simulink model "slexCreditRatingClassificationEnsemblePredictExample"  (R2021a)
settings: Solver=FixedStepDiscrete  StartTime=0.0  StopTime=creditRatingInput.time(end)  RelTol=1e-3
PreLoadFcn:
  | tbl = readtable('CreditRating_Historical.dat');
  | 
  | d = dummyvar(tbl.Industry);
  | X = [table2array(tbl(:,2:6)) d];
  | Y = tbl.Rating;
  | 
  | prsntX = X(1:3000,:);
  | prsntY = Y(1:3000);
  | ftrX = X(3001:end,:);
  | ftrY = Y(3001:end);
  | 
  | rng('default')
  | t = templateTree('Reproducible',true,'MinLeafSize',5);
  | ensMdl = fitcensemble(prsntX,prsntY, ...
  |     'Learners',t, ...
  |     'ClassNames',{'AAA' 'AA' 'A' 'BBB' 'BB' 'B' 'CCC'}, ...
  |     'Method','Bag', ...
  |     'NumLearningCycles',499');
  | 
  | creditRatingInput.time = (0:931)';
  | creditRatingInput.signals(1).values = ftrX;
  | creditRatingInput.signals(1).dimensions = size(ftrX,2);
libraries: statsLibrary x1
settings Model: Creator=The MathWorks, Inc.  LastModifiedBy=The MathWorks, Inc.
settings SolverCC: AlgebraicLoopSolver=TrustRegion
settings DataIOCC: ExternalInput=creditRatingInput  LoadExternalInput=on
settings DebuggingCC: SFMachineParentedDataDiag=warning

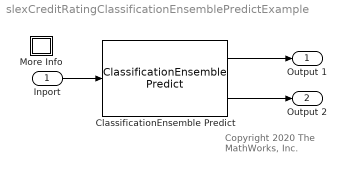
== system slexCreditRatingClassificationEnsemblePredictExample ==
  note: Copyright 2020 The MathWorks, Inc.
  Inport : Inport  PortDimensions=17
  ClassificationEnsemble Predict : statsLibrary/Classification/ClassificationEnsemble Predict  TrainedLearner=ensMdl  ShowOutputScore=on  LabelOutMin=[]  LabelOutMax=[]  ScoreOutMin=[]  ScoreOutMax=[]  RawScoreOutMin=[]  RawScoreOutMax=[]  WeakLearnerOutMin=[]  WeakLearnerOutMax=[]  StoredEnumName=ensMdl_enumLabels
      settings: SourceProductBaseCode=ST
  More Info : Subsystem
      settings: OpenFcn=showExample('stats/PredictClassLabelsClassificationEnsemblePredictBlockExample')
      mask Display: disp('?')
  Output 1 : Outport
  Output 2 : Outport  Port=2
  wires:
  Inport/1 -> ClassificationEnsemble Predict/1
  ClassificationEnsemble Predict/1 -> Output 1/1
  ClassificationEnsemble Predict/2 -> Output 2/1

== system slexCreditRatingClassificationEnsemblePredictExample/More Info ==
